simulink model "DT_DSM_CIFF_MODEL_SECOND_ORDER_OSR_2048"  (R2025b)
settings: Solver=VariableStepAuto  StartTime=0.0  StopTime=1  RelTol=1e-3
libraries: simulink_extras x1
settings Model: Creator=Team_33  LastModifiedBy=k2vas

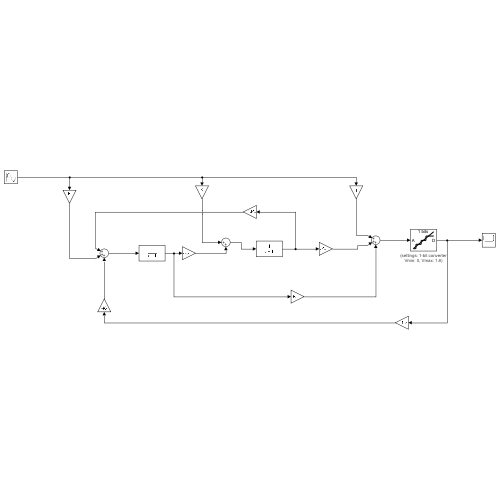
[thumbnail: Simulink's stored preview of the top-level diagram]
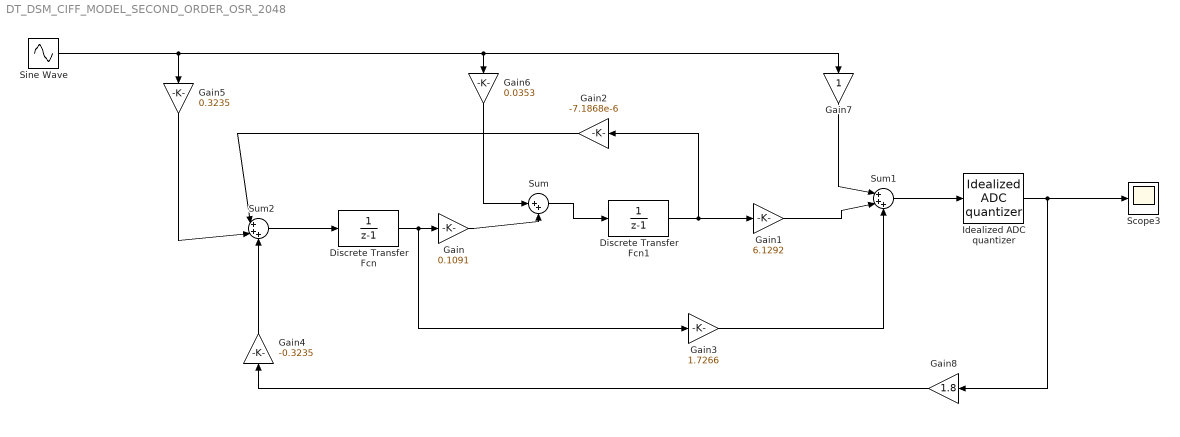
== system DT_DSM_CIFF_MODEL_SECOND_ORDER_OSR_2048 ==
  Discrete Transfer Fcn : DiscreteTransferFcn  Denominator=[1 -1]
  Discrete Transfer Fcn1 : DiscreteTransferFcn  Denominator=[1 -1]
  Gain : Gain  Gain=0.1091
  Gain1 : Gain  Gain=6.1292
  Gain2 : Gain  Gain=-7.1868e-6
  Gain3 : Gain  Gain=1.7266
  Gain4 : Gain  Gain=-0.3235
  Gain5 : Gain  Gain=0.3235
  Gain6 : Gain  Gain=0.0353
  Gain7 : Gain
  Gain8 : Gain  Gain=1.8
  Idealized ADC quantizer : simulink_extras/Additional Discrete/Idealized ADC quantizer  NumberOfConverterBits=1  Vmin=0  Vmax=1.8  OutputDataType=int16  OutputNegativeValues=off
  Scope3 : Scope
      settings: ActiveDisplayYMinimum=1.03994  ActiveDisplayYMaximum=1.04051  DataLoggingVariableName=output_data  DataLoggingSaveFormat=Array
  Sine Wave : Sin  Amplitude=0.5  Bias=0.9  Frequency=(2000*2048)*(2*pi*127)/(32768*32)  SampleTime=1/(2000*2048)
  Sum : Sum  Inputs=|++
  Sum1 : Sum  Inputs=|+++
  Sum2 : Sum  Inputs=|+++
  wires:
  Gain/1 -> Sum/2
  Gain5/1 -> Sum2/2
  Gain7/1 -> Sum1/1
  Gain1/1 -> Sum1/2
  Discrete Transfer Fcn1/1 -> Gain2/1, Gain1/1
  Gain2/1 -> Sum2/1
  Gain6/1 -> Sum/1
  Sine Wave/1 -> Gain7/1, Gain6/1, Gain5/1
  Sum/1 -> Discrete Transfer Fcn1/1
  Gain3/1 -> Sum1/3
  Gain4/1 -> Sum2/3
  Sum1/1 -> Idealized ADC quantizer/1
  Discrete Transfer Fcn/1 -> Gain3/1, Gain/1
  Idealized ADC quantizer/1 -> Scope3/1, Gain8/1
  Sum2/1 -> Discrete Transfer Fcn/1
  Gain8/1 -> Gain4/1
